simulink model "innerModel"  (Simulink 9.0)
settings: Solver=VariableStepAuto  StartTime=0.0  StopTime=10.0  RelTol=1e-3
values from neighbouring files (symbols this model uses):
  m = 1    [Controllability.m]    (also in IdealParameter.m = 2.5; ParLuk11.m = 0.6; Parameter.m = 4.85; ParameterIdeal.m = 4.85)
libraries: vrlib x2
settings Model: SuppressorTable=22 serialization::archive 11 0 6 0 0 0 11 0  Creator=jan  LastModifiedBy=jan
settings DataIOCC: SaveFormat=Dataset
settings OptimizationCC: LifeSpan=auto
settings DebuggingCC: UnderspecifiedInitializationDetection=Simplified  MergeDetectMultiDrivingBlocksExec=error  SFUnexpectedBacktrackingDiag=error  SFNoUnconditionalDefaultTransitionDiag=error  SFExecutionAtInitializationDiag=warning
settings HardwareCC: ProdBitPerPointer=64  ProdBitPerSizeT=64  ProdBitPerPtrDiffT=64  ProdLargestAtomicFloat=Float  ProdIntDivRoundTo=Zero  ProdEndianess=LittleEndian  ProdWordSize=64  ProdHWDeviceType=Intel->x86-64 (Windows64)
settings ModelReferenceCC: PropagateSignalLabelsOutOfModel=on
settings CodeAppCC: StateflowObjectComments=off
settings GRTTargetCC: TargetLangStandard=C99 (ISO)
settings ConfigComp: CovMetricSettings=dwe  CovHtmlReporting=off  CovSaveCumulativeToWorkspaceVar=off  CovSaveSingleToWorkspaceVar=off  CovExternalEMLEnable=on

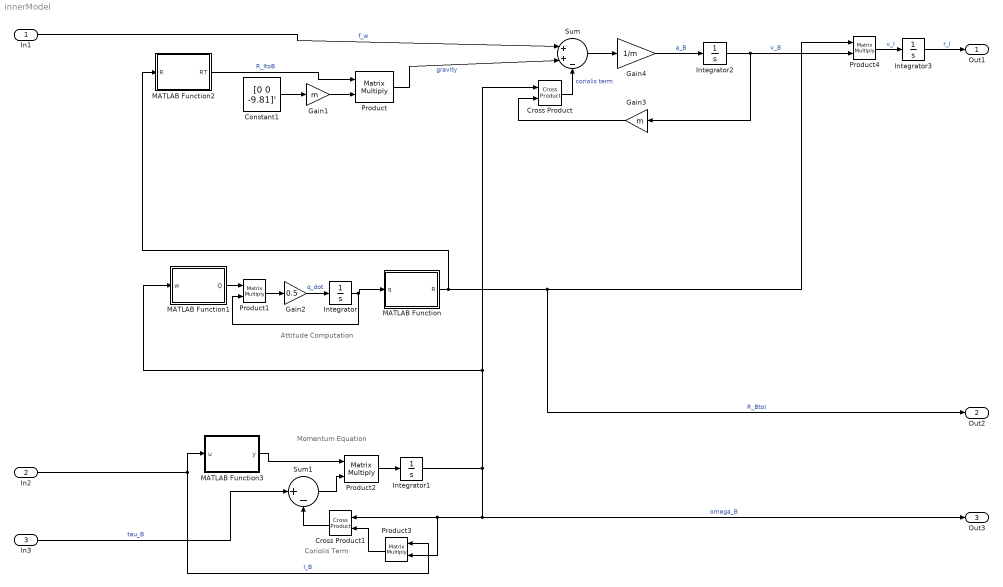
== system innerModel ==
  note: Attitude Computation
  note: Momentum Equation
  note: Coriolis Term
  In1 : Inport
  In2 : Inport  Port=2
  In3 : Inport  Port=3
  Constant1 : Constant  Value=[0 0 -9.81]'  VectorParams1D=off
  Cross Product : vrlib/Utilities/Cross Product
      settings: SourceProductBaseCode=VR
  Cross Product1 : vrlib/Utilities/Cross Product
      settings: SourceProductBaseCode=VR
  Gain1 : Gain  Gain=m
  Gain2 : Gain  Gain=0.5
  Gain3 : Gain  Gain=m
  Gain4 : Gain  Gain=1/m
  Integrator : Integrator  InitialCondition=[0 0 0 1]
  Integrator1 : Integrator  InitialCondition=[0 0 0]
  Integrator2 : Integrator
  Integrator3 : Integrator  InitialCondition=[0 0 0]'
  MATLAB Function : MATLAB Function  TreatAsAtomicUnit=on
  MATLAB Function1 : MATLAB Function  TreatAsAtomicUnit=on
  MATLAB Function2 : MATLAB Function  TreatAsAtomicUnit=on
  MATLAB Function3 : MATLAB Function  TreatAsAtomicUnit=on
  Product{,1..4} (5 alike) : Product  Multiplication=Matrix(*)
  Sum : Sum  Inputs=|++-
  Sum1 : Sum  Inputs=|+-
  Out1 : Outport
  Out2 : Outport  Port=2
  Out3 : Outport  Port=3
  wires:
  Product1/1 -> Gain2/1
  Product3/1 -> Cross Product1/2
  MATLAB Function2/1(RT) -> Product/1  "R_ItoB"
  MATLAB Function/1(R) -> MATLAB Function2/1(R), Out2/1, Product4/1  "R_BtoI"
  Cross Product1/1 -> Sum1/2
  Gain2/1 -> Integrator/1  "q_dot"
  Product/1 -> Sum/2  "gravity"
  Sum1/1 -> Product2/2
  Gain1/1 -> Product/2
  Constant1/1 -> Gain1/1
  Integrator/1 -> Product1/2, MATLAB Function/1(q)
  MATLAB Function3/1(y) -> Product2/1
  MATLAB Function1/1(Q) -> Product1/1
  In2/1 -> Product3/1, MATLAB Function3/1(u)  "I_B"
  Product2/1 -> Integrator1/1
  In3/1 -> Sum1/1  "tau_B"
  Gain3/1 -> Cross Product/2
  Integrator1/1 -> Out3/1, Product3/2, Cross Product1/1, MATLAB Function1/1(w), Cross Product/1  "omega_B"
  In1/1 -> Sum/1  "f_w"
  Integrator2/1 -> Product4/2, Gain3/1  "v_B"
  Cross Product/1 -> Sum/3  "coriolis term"
  Sum/1 -> Gain4/1
  Product4/1 -> Integrator3/1  "v_I"
  Gain4/1 -> Integrator2/1  "a_B"
  Integrator3/1 -> Out1/1  "r_I"

== matlab function MATLAB Function1 ==
  data: w input double; Q output double
function Q = omegaSkew(w)
%#codegen

Q = [0 w(3) -w(2) w(1);
    -w(3) 0 w(1) w(2);
    w(2) -w(1) 0 w(3);
    -w(1) -w(2) -w(3) 0];

== matlab function MATLAB Function ==
  data: q input double; R output double
function R = Quat2R(q)
% compute R from quaternion input

R = [q(1)^2 - q(2)^2 - q(3)^2 + q(4)^2,  2*(q(1)*q(2) - q(3)*q(4)),          2*(q(1)*q(3) + q(2)*q(4));
     2*(q(1)*q(2) + q(3)*q(4)),         -q(1)^2 + q(2)^2 - q(3)^2 + q(4)^2,  2*(q(2)*q(3) - q(1)*q(4));
     2*(q(1)*q(3) - q(2)*q(4)),          2*(q(2)*q(3) + q(1)*q(4)),         -q(1)^2 - q(2)^2 + q(3)^2 + q(4)^2];

== matlab function MATLAB Function2 ==
  data: R input double; RT output double
function RT = transpose(R)
%#codegen

RT = R';

== matlab function MATLAB Function3 ==
  data: u input double; y output double
function y = inverse(u)
%#codegen

y = inv(u);
